simulink model "mup_rmpcblock_soft_con_demo_model_R2011b"  (Simulink 7.8)
settings: Solver=ode4  StartTime=0.0  StopTime=25  RelTol=1e-3
values from neighbouring files (symbols this model uses):
  nu = size(B{1},2)    [mup_rmpcblock_soft_con_demo.m]
  nx = size(A{1},2)    [mup_rmpcblock_soft_con_demo.m]
  ts = 1    [mup_rmpcblock_soft_con_demo.m]
  u_max = [10]    [mup_rmpc_soft_con_demo.m]    (also in mup_rmpcblock_soft_con_demo.m)
  u_sl = 0.4    [mup_rmpc_soft_con_demo.m]    (also in mup_rmpcblock_soft_con_demo.m = 0.3; mup_soft_con_param.m = param.u_sl)
  us = [0;0]    [mup_rmpcblock_soft_con_demo.m]
  Wu = eye(1)    [mup_rmpc_soft_con_demo.m]    (also in mup_rmpcblock_soft_con_demo.m)
  Wx = eye(2)    [mup_rmpc_soft_con_demo.m]    (also in mup_rmpcblock_soft_con_demo.m)
  x0 = [3;0]    [mup_rmpc_soft_con_demo.m]    (also in mup_rmpcblock_soft_con_demo.m)
  x_max = [10;10]    [mup_rmpc_soft_con_demo.m]    (also in mup_rmpcblock_soft_con_demo.m)
  xs = [0;0]    [mup_rmpcblock_soft_con_demo.m]
  y_sl = [1;0.5]    [mup_rmpc_soft_con_demo.m]    (also in mup_rmpcblock_soft_con_demo.m; mup_soft_con_param.m = param.y_sl)
undefined symbols (not defined in the file or in its folder): A, B, C, params
settings Model: Creator=oravec  LastModifiedBy=oravec
settings DataIOCC: SignalLoggingSaveFormat=Dataset
settings OptimizationCC: ExpressionDepthLimit=128
settings CodeAppCC: CustomSymbolStrType=$N$R$M_T
settings GRTTargetCC: TargetFunctionLibrary=C89/C90 (ANSI)

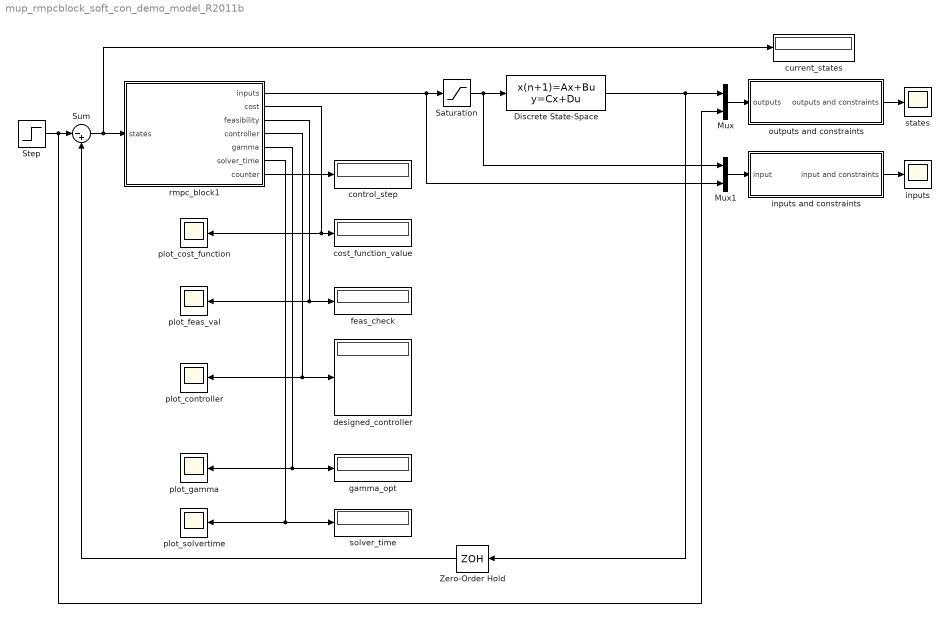
== system mup_rmpcblock_soft_con_demo_model_R2011b ==
  Discrete State-Space : DiscreteStateSpace  A=A{vtx}  B=B{vtx}  C=C{vtx}  D=zeros(nx,nu)  X0=x0  SampleTime=ts
  Mux : Mux  Inputs=2
  Mux1 : Mux  Inputs=2
  Saturation : Saturate  UpperLimit=u_max  LowerLimit=-u_max
  Step : Step  Time=0  Before=zeros(nx,1)  After=zeros(nx,1)  SampleTime=0
  Sum : Sum  Inputs=|-+
  Zero-Order Hold : ZeroOrderHold  SampleTime=ts
  control_step : Display
  cost_function_value : Display
  current_states : Display
  designed_controller : Display
  feas_check : Display
  gamma_opt : Display
  inputs : Scope
      settings: YMin=-1.1  YMax=0.3  SaveName=data_u
  inputs and constraints : Subsystem  mask{us=us, u_max=u_max, u_sl=u_sl}
      mask prompts: us "Steady State Input: us"; u_max "Hard Constraints: u_max"; u_sl "Soft Constraints: u_sl"
  outputs and constraints : Subsystem  mask{xs=xs, x_max=x_max, y_sl=y_sl}
      mask prompts: xs "System Steady State: xs"; x_max "Hard Constraints: x_max"; y_sl "Soft Constraints: y_sl"
  plot_controller : Scope
      settings: YMin=0  YMax=2  SaveName=f_des
  plot_cost_function : Scope
      settings: YMin=0  YMax=2  SaveName=cost
  plot_feas_val : Scope
      settings: YMin=0  YMax=2  SaveName=feas_val
  plot_gamma : Scope
      settings: YMin=0  YMax=2  SaveName=gamma_val
  plot_solvertime : Scope
      settings: YMin=0  YMax=2  SaveName=solvertime_val
  rmpc_block1 : Subsystem  Tag=rmpc_tag  mask(RMPC){rmpc_method=Kothare et al. (1996) - Soft-Con, opt_type=initial, chk_feas=on, feas_toler=-1e-6, x0=x0, A=A, B=B, C=C, Ts=ts, Wu=Wu, Wx=Wx, u_max=u_max, x_max=x_max, param=params, chk_soft_con=on, u_sl=params.u_sl, y_sl=params.y_sl, Wsu=params.Wsu, Wsy=params.Wsy, solver=MOSEK, vbs=Normal, vbsy=Silent}
      mask prompts: rmpc_method "Robust MPC Approach:"; opt_type "Optimization Problem Design:"; chk_feas "Feasibility Check (Disable to speed up control)"; feas_toler "Feasibility Tolerance: (Relevant, if Feasibility Check is enable)"; x0 "Initial Conditions of System States: x0"; A "System State Matrix: A"; B "System Input Matrix: B"; C "System Output Matrix: C"; Ts "Sampling Time: Ts"; Wu "Cost Function Weight of Inputs: Wu"; Wx "Cost Function Weight of States: Wx"; u_max "Symmetric Constraint on Control Input: u_max"; x_max "Symmetric Constraint on System Outputs: y_max"; param "Parameters:"; chk_soft_con "Consider Soft Constraints: chk_soft_con"; u_sl "Soft-constrained Control Inputs: u_sl"; y_sl "Soft-constrained System Outputs: y_sl"; Wsu "Weight of Soft-constrained Control Inputs: Wsu"; Wsy "Weight of Soft-constrained System Outputs: Wsy"; solver "SDP Solver:"; vbs "Verbose Mode:"; vbsy "YALMIP Verbose Mode:"
      mask help: Computes on-line robust MPC control inputs for a given state.
      mask init:
      | mup_rmpc_data
      | mup_rmpc_init(design,model,setup)
      mask Help: eval('mup_rmpc_help')
      mask StyleString: popup(Kothare et al. (1996)|Cuzzola et al. (2002)|Mao (2003)|Wan et al. (2003)|Cao et al. (2005)|Ding et al. (2007)|Li et al. (2008)|Huang et al. (2011)|Zhang et al. (2013)|NSO and ACIS|NSO and WACIS|NSO and SDLF|PDLF and ACIS|PDLF and WACIS|Kothare et al. (1996) - Soft-Con|Wan et al. (2003) - Soft-Con|Cao et al. (2005) - Soft-Con|NSO and ACIS - Soft-Con),popup(initial|reformulation),checkbox,edit,edit,edit,edit,edit,edit,edit,edit,edit,edit,edit,checkbox,edit,edit,edit,edit,popup(CSDP|DSDP|LMILAB|LOGDETPPA|MOSEK|PENBMI|PENLAB|PENSDP|SDPA|SDPLR|SDPT3|SDPNAL|SEDUMI),popup(Normal|Silent|Loud),popup(Silent|Loud)
      mask TabNameString: Robust MPC Configuration,Robust MPC Configuration,Robust MPC Configuration,Robust MPC Configuration,Robust MPC Configuration,Robust MPC Configuration,Robust MPC Configuration,Robust MPC Configuration,Robust MPC Configuration,Robust MPC Configuration,Robust MPC Configuration,Robust MPC Configuration,Robust MPC Configuration,Robust MPC Configuration,SOFT-CON,SOFT-CON,SOFT-CON,SOFT-CON,SOFT-CON,Setup,Setup,Setup
      mask Display:
      | disp('RMPC')
      | port_label('input',1,'states')
      | port_label('output',1,'inputs')
      | port_label('output',2,'cost')
      | port_label('output',3,'feasibility')
      | port_label('output',4,'controller')
      | port_label('output',5,'gamma')
      | port_label('output',6,'solver_time')
      | port_label('output',7,'counter')
  solver_time : Display
  states : Scope
      settings: YMin=-0.02  YMax=0.1  SaveName=data_x
  wires:
  rmpc_block1/2(cost) -> plot_cost_function/1, cost_function_value/1
  Sum/1 -> current_states/1, rmpc_block1/1(states)
  Step/1 -> Mux/2, Sum/1
  Discrete State-Space/1 -> Mux/1, Zero-Order Hold/1
  Zero-Order Hold/1 -> Sum/2
  Mux/1 -> outputs and constraints/1(outputs)
  Saturation/1 -> Discrete State-Space/1, Mux1/1
  rmpc_block1/1(inputs) -> Saturation/1, Mux1/2
  Mux1/1 -> inputs and constraints/1(input)
  rmpc_block1/7(counter) -> control_step/1
  rmpc_block1/3(feasibility) -> feas_check/1, plot_feas_val/1
  rmpc_block1/4(controller) -> designed_controller/1, plot_controller/1
  rmpc_block1/5(gamma) -> gamma_opt/1, plot_gamma/1
  rmpc_block1/6(solver_time) -> plot_solvertime/1, solver_time/1
  inputs and constraints/1(input and constraints) -> inputs/1
  outputs and constraints/1(outputs and constraints) -> states/1

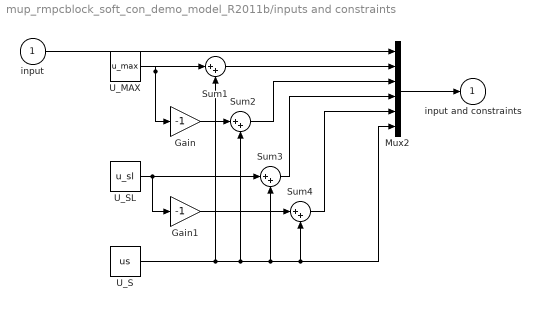
== system mup_rmpcblock_soft_con_demo_model_R2011b/inputs and constraints ==
  input : Inport
  Gain : Gain  Gain=-1
  Gain1 : Gain  Gain=-1
  Mux2 : Mux  Inputs=6
  Sum{1..4} (4 alike) : Sum  Inputs=|++
  U_MAX : Constant  Value=u_max
  U_S : Constant  Value=us
  U_SL : Constant  Value=u_sl
  input and constraints : Outport
  wires:
  input/1 -> Mux2/1
  U_S/1 -> Sum1/2, Sum4/2, Mux2/6, Sum3/2, Sum2/2
  Sum3/1 -> Mux2/4
  Gain1/1 -> Sum4/1
  Sum4/1 -> Mux2/5
  U_SL/1 -> Gain1/1, Sum3/1
  Sum2/1 -> Mux2/3
  Mux2/1 -> input and constraints/1
  Gain/1 -> Sum2/1
  Sum1/1 -> Mux2/2
  U_MAX/1 -> Gain/1, Sum1/1

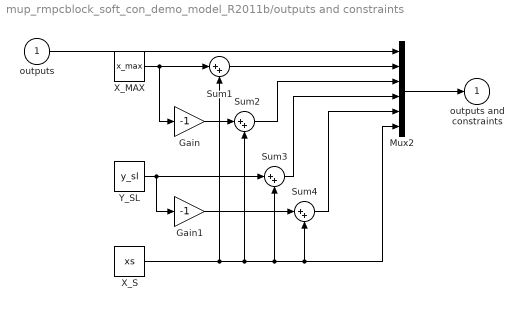
== system mup_rmpcblock_soft_con_demo_model_R2011b/outputs and constraints ==
  outputs : Inport
  Gain : Gain  Gain=-1
  Gain1 : Gain  Gain=-1
  Mux2 : Mux  Inputs=6
  Sum{1..4} (4 alike) : Sum  Inputs=|++
  X_MAX : Constant  Value=x_max
  X_S : Constant  Value=xs
  Y_SL : Constant  Value=y_sl
  outputs and constraints : Outport
  wires:
  outputs/1 -> Mux2/1
  X_S/1 -> Sum1/2, Sum4/2, Mux2/6, Sum3/2, Sum2/2
  Sum3/1 -> Mux2/4
  Gain1/1 -> Sum4/1
  Sum4/1 -> Mux2/5
  Y_SL/1 -> Gain1/1, Sum3/1
  Sum2/1 -> Mux2/3
  Mux2/1 -> outputs and constraints/1
  Gain/1 -> Sum2/1
  Sum1/1 -> Mux2/2
  X_MAX/1 -> Gain/1, Sum1/1

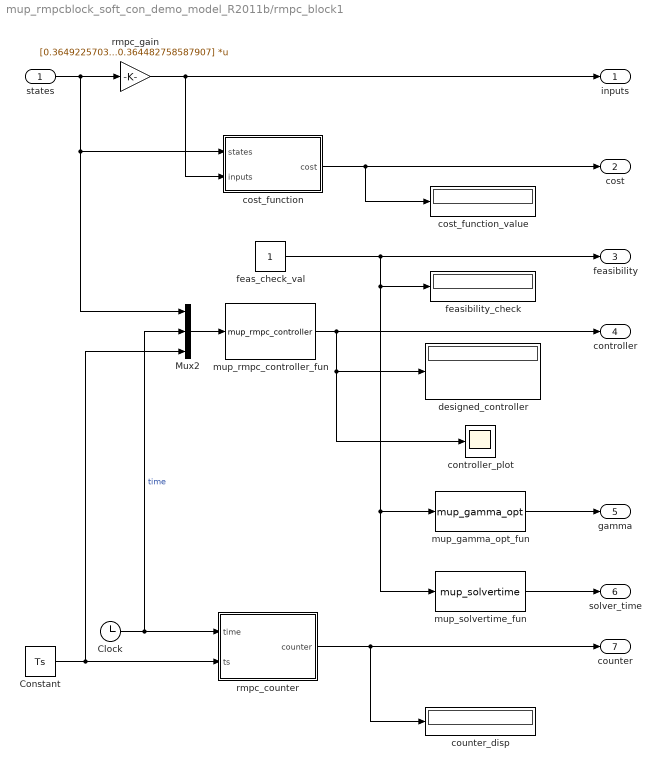
== system mup_rmpcblock_soft_con_demo_model_R2011b/rmpc_block1 ==
  states : Inport
  Clock : Clock
  Constant : Constant  Value=Ts
  Mux2 : Mux  Inputs=3
  controller_plot : Scope
      settings: TimeRange=50  SaveName=rmpc_designed_controller  MaxDataPoints=50000
  cost_function : Subsystem
  cost_function_value : Display
  counter_disp : Display
  designed_controller : Display
  feas_check_val : Constant
  feasibility_check : Display
  mup_gamma_opt_fun : MATLABFcn  MATLABFcn=mup_gamma_opt
  mup_rmpc_controller_fun : MATLABFcn  MATLABFcn=mup_rmpc_controller
  mup_solvertime_fun : MATLABFcn  MATLABFcn=mup_solvertime
  rmpc_counter : Subsystem
  rmpc_gain : Gain  Tag=rmpc_gain_2013_3_25_11_17_59.8099  Gain=[0.364922570332082,0.364482758587907]  Multiplication=Matrix(K*u)
  inputs : Outport
  cost : Outport  Port=2
  feasibility : Outport  Port=3
  controller : Outport  Port=4
  gamma : Outport  Port=5
  solver_time : Outport  Port=6
  counter : Outport  Port=7
  wires:
  rmpc_gain/1 -> inputs/1, cost_function/2(inputs)
  states/1 -> rmpc_gain/1, Mux2/1, cost_function/1(states)
  cost_function/1(cost) -> cost_function_value/1, cost/1
  rmpc_counter/1(counter) -> counter_disp/1, counter/1
  Clock/1 -> rmpc_counter/1(time), Mux2/2  "time"
  Constant/1 -> rmpc_counter/2(ts), Mux2/3
  feas_check_val/1 -> feasibility/1, mup_solvertime_fun/1, mup_gamma_opt_fun/1, feasibility_check/1
  mup_rmpc_controller_fun/1 -> controller/1, designed_controller/1, controller_plot/1
  Mux2/1 -> mup_rmpc_controller_fun/1
  mup_gamma_opt_fun/1 -> gamma/1
  mup_solvertime_fun/1 -> solver_time/1

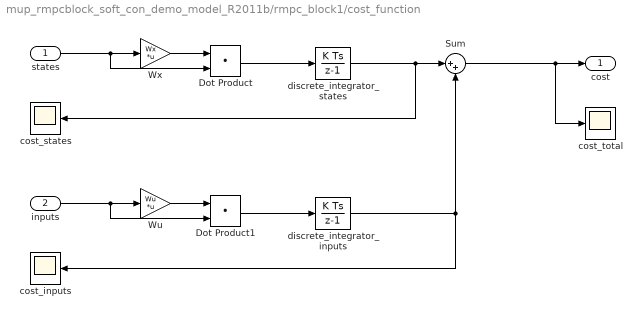
== system mup_rmpcblock_soft_con_demo_model_R2011b/rmpc_block1/cost_function ==
  states : Inport
  inputs : Inport  Port=2
  Dot Product : DotProduct  InputSameDT=on  OutDataTypeStr=Inherit: Inherit via internal rule
  Dot Product1 : DotProduct  InputSameDT=on  OutDataTypeStr=Inherit: Inherit via internal rule
  Sum : Sum  Inputs=|++
  Wu : Gain  Gain=Wu  Multiplication=Matrix(K*u)
  Wx : Gain  Gain=Wx  Multiplication=Matrix(K*u)
  cost_inputs : Scope
  cost_states : Scope
      settings: SaveName=ScopeData2
  cost_total : Scope
      settings: SaveName=ScopeData3
  discrete_integrator_inputs : DiscreteIntegrator  SampleTime=Ts
  discrete_integrator_states : DiscreteIntegrator  SampleTime=Ts
  cost : Outport
  wires:
  Dot Product1/1 -> discrete_integrator_inputs/1
  Wu/1 -> Dot Product1/1
  Dot Product/1 -> discrete_integrator_states/1
  Wx/1 -> Dot Product/1
  states/1 -> Dot Product/2, Wx/1
  inputs/1 -> Dot Product1/2, Wu/1
  Sum/1 -> cost/1, cost_total/1
  discrete_integrator_states/1 -> Sum/1, cost_states/1
  discrete_integrator_inputs/1 -> Sum/2, cost_inputs/1

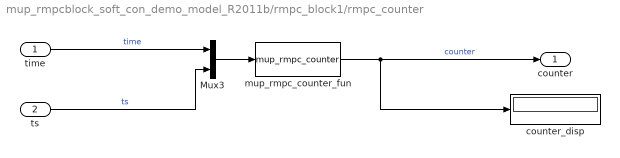
== system mup_rmpcblock_soft_con_demo_model_R2011b/rmpc_block1/rmpc_counter ==
  time : Inport
  ts : Inport  Port=2
  Mux3 : Mux  Inputs=2
  counter_disp : Display
  mup_rmpc_counter_fun : MATLABFcn  MATLABFcn=mup_rmpc_counter
  counter : Outport
  wires:
  mup_rmpc_counter_fun/1 -> counter/1, counter_disp/1  "counter"
  ts/1 -> Mux3/2  "ts"
  time/1 -> Mux3/1  "time"
  Mux3/1 -> mup_rmpc_counter_fun/1
